simulink model "power_battery"  (R2013b)
settings: Solver=ode23tb  StartTime=0.0  StopTime=3600  MaxStep=0.1  RelTol=1e-4
undefined symbols (not defined in the file): Hydride, Metal, Nickel
libraries: powerlib x3, electricdrivelib x1
Description:
  | Copyright 2008-2013 The MathWorks, Inc.
settings Model: Creator=MathWorks  LastModifiedBy=dmeissne
settings DataIOCC: SignalLoggingSaveFormat=ModelDataLogs
settings OptimizationCC: ExpressionDepthLimit=2147483647  InitFltsAndDblsToZero=on
settings DebuggingCC: SignalResolutionControl=TryResolveAllWithWarning  FcnCallInpInsideContextMsg=UseLocalSettings  StateNameClashWarn=warning
settings GRTTargetCC: CombineOutputUpdateFcns=off  GRTInterface=on

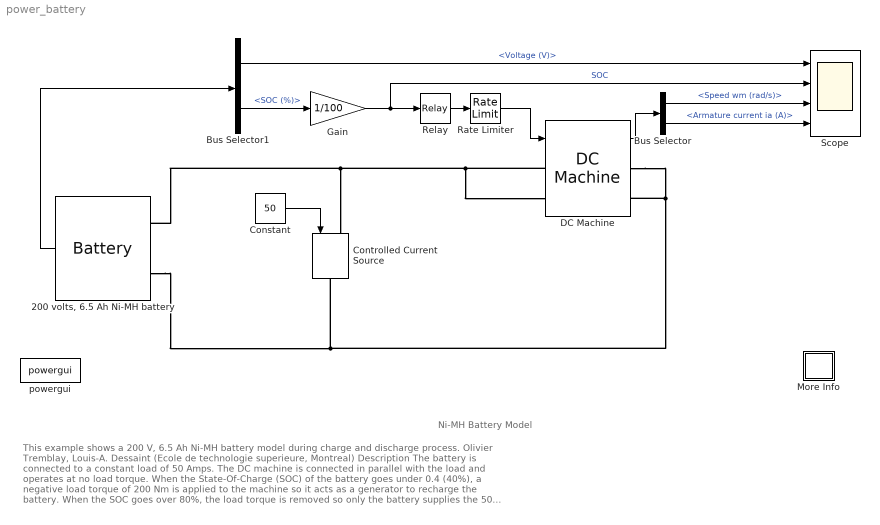
== system power_battery ==
  note: This example shows a 200 V, 6.5 Ah Ni-MH battery model during charge and discharge process.  Olivier Tremblay, Louis-A. Dessaint (Ecole de technologie superieure, Montreal)
      |
      | Description
      |
      | The battery is connected to a constant load of 50 Amps. The DC machine is connected in parallel with the load and operates at no load torque.
      | When the State-Of-Charge (SOC) of the battery goes under 0.4 (40%), a negative load torque of 200 Nm is applied to the machine so it acts as
      | a generator to recharge the battery. When the SOC goes over 80%, the load torque is removed so only the battery supplies the 50 amps load.
      |
      | Battery voltage, SOC, Motor speed and Motor current signals are available at the output of the block.
      |
      | Simulation
      |
      | At t = 0 s, the DC machine is started with the battery power. The speed increases to 120 rad/s. The battery is also discharged by the constant
      | DC load of 50 amps. At t = 280 s, the SOC drops under 40%. A mechanical torque of -200 Nm is applied to the machine so it acts as a generator
      | and provides a current of 100 amps. Hence, 50 amps goes to the load and 50 amps goes to recharge the battery. At t = 500 s, the SOC goes over 80%.
      | The mechanical torque is removed and the machine operates free. And the cycle restarts.
      |
      | References
      |
      | 1. O. Tremblay, L.-A. Dessaint, A.-I. Dekkiche, ?A Generic Battery Model for the Dynamic Simulation of Hybrid Electric Vehicles?, 2007 IEEE
      |  Vehicle Power and Propulsion Conference, September 9-13, 2007 ? Arlington/Texas, USA
  note: Ni-MH Battery Model
  "200 volts, 6.5 Ah Ni-MH battery " : electricdrivelib/Extra Sources/Battery  BatType=Nickel-Metal-Hydride  ShowDetailedParameters=off  NomV=200  NomQ=6.5  SOC=100  PresetModel=on  MaxQ=7  FullV=235.5932  Dis_rate=1.3  R=0.30769  Normal_OP=6.25  expZone="[216.9492           1.3]"  Dis_Char=off  current=50  Units=Ampere-hour  Batt_Tr=30
  Bus Selector : BusSelector  OutputSignals=Speed wm (rad/s),Armature current ia (A)
  Bus Selector1 : BusSelector  OutputSignals=Voltage (V),SOC (%)
  Constant : Constant  Value=50
  Controlled Current Source : powerlib/Electrical Sources/Controlled Current Source  Initialize=on  Source_Type=AC  Amplitude=0  Phase=0  Frequency=0  Measurements=None
  DC Machine : powerlib/Machines/DC Machine  PresetModel=No  MechanicalLoad=Torque TL  FieldType=Wound  ShowDetailedParameters=on  RLa=[0.4832 0.006763]  RLf=[84.91 13.39]  Laf=0.7096  MachineConstant=Torque constant (N.m/A)  Ke=1.8  Kt=1.8  J=0.2053  Bm=0.007032  Tf=0  w0=0  Ifinit=0  TsPowergui=0  TsBlock=-1
  Gain : Gain  Gain=1/100
  More Info : Subsystem
      settings: OpenFcn=showdemo(bdroot(gcb))
      mask Display: disp('?')
  Rate Limiter : RateLimiter  RisingSlewLimit=100  FallingSlewLimit=-100  SampleTimeMode=inherited
  Relay : Relay  OnSwitchValue=0.8  OffSwitchValue=0.4  OnOutputValue=0  OffOutputValue=-200
  Scope : Scope  NumInputPorts=4
      settings: TimeRange=3600  YMin=100~0~-5.41510190224349e-025~-200  YMax=300~1~200~400
  powergui : powerlib/powergui  SimulationMode=Continuous  SolverType=Tustin  SampleTime=0.001  frequency=60  SPID=off  DisableSnubberDevices=off  DisableRonSwitches=off  DisableVfSwitches=off  SwTol=0  Interpol=off  DisplayEquations=off  frequencyindice=0  Pbase=100e6  ErrMax=1e-4  Iterations=50  UnitsV=kV  UnitsW=MW  FunctionMessages=off  echomessages=off  HookPort=off  EnableUseOfTLC=off  x0status=blocks  RestoreLinks=warning  ResistiveCurrentMeasurement=off  Frange=[0:2:500]  Ylog=off  Xlog=on  ShowGrid=off  save=off  variable=ZData  ZoomFFT=on  StartTime=0.0  cycles=1  DisplayStyle=1  fundamental=60  FreqAxis=off  MaxFrequency=1000  frequencyindicesteady=1  RmsSteady=1  display=off  Ts=0  methode=off
  wires:
  DC Machine/1 -> Bus Selector/1
  Constant/1 -> Controlled Current Source/1
  Relay/1 -> Rate Limiter/1
  Bus Selector/1 -> Scope/3  "<Speed wm (rad/s)>"
  Bus Selector/2 -> Scope/4  "<Armature current ia (A)>"
  Rate Limiter/1 -> DC Machine/1
  "200 volts, 6.5 Ah Ni-MH battery "/1 -> Bus Selector1/1
  Bus Selector1/2 -> Gain/1  "<SOC (%)>"
  Gain/1 -> Relay/1, Scope/2  "SOC"
  Bus Selector1/1 -> Scope/1  "<Voltage (V)>"
  connections:
  "200 volts, 6.5 Ah Ni-MH battery "/LConn2 -- DC Machine/RConn1 -- DC Machine/RConn2 -- Controlled Current Source/RConn1
  "200 volts, 6.5 Ah Ni-MH battery "/LConn1 -- DC Machine/LConn1 -- DC Machine/LConn2 -- Controlled Current Source/LConn1

== system power_battery/More Info ==
